simulink library "wcdma_lib"  (Simulink 6.0)
settings: Solver=ode45  SolverMode=SingleTasking  StartTime=0.0  StopTime=10.0  RelTol=1e-3
values from neighbouring files (symbols this model uses):
  allocationssc = [1 1 1 1 1 1 1 1 1 1 1 1 ... (960 elements, 64x15)]    [wcdma_allocationssc.mat]
  crcSize = str2num(Vals{idxCrcSize})    [wcdma_initmaskphlayer.m]    (also in wcdma_loadinitmuxandcoding.m = [16 12]; wcdma_loadinitphlayer.m = [16 12])
  errorCorr = (errorCorr>2)*2 + (errorCorr<3).*errorCorr    [wcdma_initmaskphlayer.m]    (also in wcdma_loadinitmuxandcoding.m = [2 2]; wcdma_loadinitphlayer.m = [2 2])
  i = [1:2:numSamp-1]'    [cdma2000_inttable.m]
  numBitsCodeWord = cond.*Zmin + not(cond).*numBitsCodeWord    [wcdma_concseg.m]    (also in wcdma_loadinitmuxandcoding.m = [260 122])
  numBitsFirstInt = numBitsRM + deltaNimax    [wcdma_initmaskphlayer.m]    (also in wcdma_loadinitmuxandcoding.m = [686 308])
  numBitsRF = numBitsFirstInt./(tti/10)    [wcdma_initmaskphlayer.m]    (also in wcdma_loadinitmuxandcoding.m = [343 77]; wcdma_loadinitphlayer.m = [343 77])
  numBitsTrCh = (trBlkSize+crcSize)*diag(numTrBlks)    [wcdma_concseg.m]    (also in wcdma_loadinitmuxandcoding.m = [260 112])
  numCodeWords = ceil(numBitsTrCh./Zmax(errorCorr+1))    [wcdma_concseg.m]    (also in wcdma_loadinitmuxandcoding.m = [1 1])
  numPadBits = (numBitsCodeWord.*numCodeWords)-numBitsTrCh    [wcdma_concseg.m]    (also in wcdma_loadinitmuxandcoding.m = [0 0])
  numPhCH = str2num(Vals{idxNumPhCH})    [wcdma_initmaskphlayer.m]    (also in wcdma_loadinitmuxandcoding.m = 1; wcdma_loadinitphlayer.m = 1)
  numTrBlks = trBlkSetSize./trBlkSize    [wcdma_concseg.m]    (also in wcdma_initmaskphlayer.m; wcdma_loadinitmuxandcoding.m = [1 1]; wcdma_loadinitphlayer.m = [1 1])
  overSampling = str2num(Vals{idxOverSampling})    [wcdma_initmaskphlayer.m]    (also in wcdma_initmaskspreadandmod.m; wcdma_loadinitphlayer.m = 8; wcdma_loadinitspreadandmod.m = 8)
  powerVector = str2num(Vals{idxPowerVector})    [wcdma_initmaskphlayer.m]    (also in wcdma_initmaskspreadandmod.m; wcdma_loadinitphlayer.m = [-5.5 -10 -15 -12 -12]; wcdma_loadinitspreadandmod.m = [-5.5 -10 -15 -12 -12])
  sprdFactor = wcdma_slotformattable(slotFormat+1,2)    [wcdma_checkparamstxant.m]    (also in wcdma_initmaskphlayer.m = slotformattable(slotFormat+1,2); wcdma_initmaskspreadandmod.m = slotformattable(slotFormat+1,2); wcdma_loadinitphlayer.m = 128; wcdma_loadinitspreadandmod.m = 128)
  tti = str2num(Vals{idxTti})    [wcdma_initmaskphlayer.m]    (also in wcdma_loadinitmuxandcoding.m = [20 40]; wcdma_loadinitphlayer.m = [20 40])
undefined symbols (not defined in the file or in its folder): hadamard, numSymbOut
libraries: wcdma_lib x122, dspsrcs4 x39, dspsigops x30, commseqgen2 x24, dspindex x20, dspbuff3 x19, dspmathops x16, simulink x10, dspsigattribs x7, commutil2 x6, dspmtrx3 x6, commblkintrlv2 x6
(part 2 of 3)

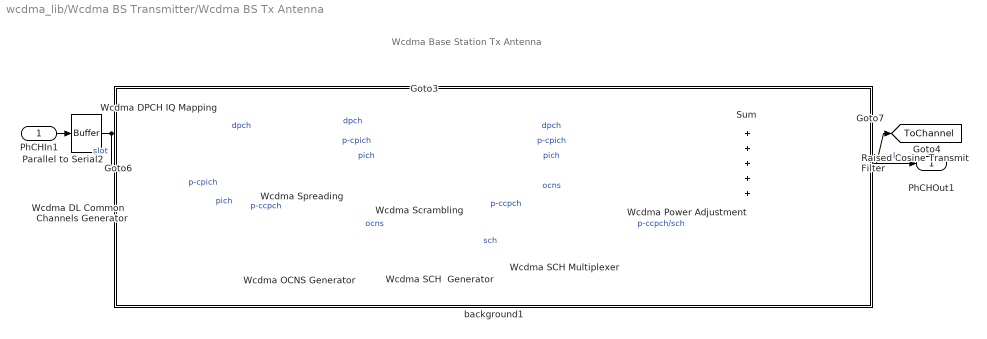
== system wcdma_lib/Wcdma BS Transmitter/Wcdma BS Tx Antenna ==
  note: Wcdma Base Station Tx Antenna
  PhCHIn1 : Inport  LatchInput=off
  Parallel to Serial2 : dspbuff3/Buffer  N=2*(numChipsOut/sprdFactor)  V=0  ic=0
  Raised Cosine Transmit Filter : commfilt2/Raised Cosine Transmit Filter  filtType=Square root  D=floor(numTapsRRC/(overSampling*2))  R=0.22  sampMode=Frame-based  N=overSampling  checkGain=User-specified  filterGain=sqrt(overSampling)  checkCoeff=off  variableName=rcTxFilt
  Sum : Sum  Inputs=+++++  SaturateOnIntegerOverflow=on  InputSameDT=on
  Wcdma DL Common  Channels Generator : wcdma_lib/Wcdma BS Transmitter/Wcdma DL Common  Channels Generator  antenna=1  numSymbOut=numChipsOut/256  st=1/15e3
  Wcdma DPCH IQ Mapping : wcdma_lib/Wcdma BS Transmitter/Wcdma DPCH IQ Mapping
  Wcdma OCNS Generator : wcdma_lib/Wcdma Sources/Wcdma OCNS Generator  sprdFactor=256  numSymbOut=numChipsOut/256  st=1/15e3
  Wcdma Power Adjustment : wcdma_lib/Wcdma BS Transmitter/Wcdma Power Adjustment  powerVector=powerVector
  Wcdma SCH  Generator : wcdma_lib/Wcdma Sources/Wcdma SCH  Generator  scrGroup=scrCode(1)  a_sch=1
  Wcdma SCH Multiplexer : wcdma_lib/Wcdma BS Transmitter/Wcdma SCH Multiplexer  numChipsOut=numChipsOut
  Wcdma Scrambling : wcdma_lib/Wcdma BS Transmitter/Wcdma Scrambling  scrCode=scrCode  numChipsOut=numChipsOut
  Wcdma Spreading : wcdma_lib/Wcdma BS Transmitter/Wcdma Spreading  sprdFactor=sprdFactor  dpchCode=dpchCode  codeVector=[0 4 1]  numChipsOut=numChipsOut
  background1 : Subsystem  EnableExecutionContextPropagation=on
      mask Display: disp('')
  PhCHOut1 : Outport
  tag scope: DPCH_Tx=global, DPCH_Tx_all=global, DPCH_Tx_sprd=global, ToChannel=global
  wires:
  Wcdma DPCH IQ Mapping/1 -> Wcdma Spreading/1  "dpch"
  Parallel to Serial2/1 -> Wcdma DPCH IQ Mapping/1, [DPCH_Tx]  "slot"
  Wcdma Spreading/3 -> Wcdma Scrambling/3  "pich"
  Wcdma Spreading/4 -> Wcdma Scrambling/4
  Wcdma DL Common  Channels Generator/1 -> Wcdma Spreading/2  "p-cpich"
  Wcdma Spreading/2 -> Wcdma Scrambling/2  "p-cpich"
  Wcdma Spreading/1 -> Wcdma Scrambling/1, [DPCH_Tx_sprd]  "dpch"
  Wcdma Scrambling/1 -> Wcdma Power Adjustment/1  "dpch"
  Wcdma Scrambling/2 -> Wcdma Power Adjustment/2  "p-cpich"
  Wcdma Scrambling/3 -> Wcdma Power Adjustment/3  "pich"
  Wcdma Power Adjustment/2 -> Sum/2
  Wcdma Power Adjustment/3 -> Sum/3
  Wcdma Power Adjustment/4 -> Sum/4
  Wcdma Power Adjustment/5 -> Sum/5
  Wcdma Scrambling/5 -> Wcdma Power Adjustment/5  "ocns"
  Wcdma Power Adjustment/1 -> Sum/1
  Wcdma SCH  Generator/1 -> Wcdma SCH Multiplexer/2  "sch"
  Wcdma Scrambling/4 -> Wcdma SCH Multiplexer/1  "p-ccpch"
  Wcdma SCH Multiplexer/1 -> Wcdma Power Adjustment/4  "p-ccpch/sch"
  Wcdma OCNS Generator/1 -> Wcdma Scrambling/5  "ocns"
  Wcdma DL Common  Channels Generator/2 -> Wcdma Spreading/3  "pich"
  Wcdma DL Common  Channels Generator/3 -> Wcdma Spreading/4  "p-ccpch"
  PhCHIn1/1 -> Parallel to Serial2/1
  Sum/1 -> [DPCH_Tx_all], Raised Cosine Transmit Filter/1
  Raised Cosine Transmit Filter/1 -> PhCHOut1/1, [ToChannel]  "l"

== system wcdma_lib/Wcdma BS Transmitter/Wcdma DL Common  Channels Generator ==
  P-CCPCH Generator : wcdma_lib/Wcdma Sources/Channel Generator  rndSeed=98765  initDelay=0  numSymbOut=numSymbOut  st=st
  P-CPICH Generator : wcdma_lib/Wcdma Sources/P-CPICH Generator  antenna=antenna  numSymbOut=numSymbOut  st=st
  PICH Generator : wcdma_lib/Wcdma Sources/Channel Generator  rndSeed=12345  initDelay=0  numSymbOut=numSymbOut  st=st
  cP-CPICH : Outport
  cPICH : Outport  Port=2
  cP-CCPCH : Outport  Port=3
  wires:
  P-CPICH Generator/1 -> cP-CPICH/1
  PICH Generator/1 -> cPICH/1
  P-CCPCH Generator/1 -> cP-CCPCH/1

== system wcdma_lib/Wcdma BS Transmitter/Wcdma DPCH IQ Mapping ==
  DPCH : Inport  LatchInput=off
  Bit to Integer Converter : commutil2/Bit to Integer Converter  nbits=2
  Data Mapper : commutil2/Data Mapper  MapMode=User Defined  M=4  MapVec=[0 3 1 2]
  QPSK Modulator Baseband : commdigbbndpm2/QPSK Modulator Baseband  InType=Integer  Enc=Binary  Ph=pi/4  numSamp=1
  cDPCH : Outport
  wires:
  Bit to Integer Converter/1 -> Data Mapper/1
  Data Mapper/1 -> QPSK Modulator Baseband/1
  DPCH/1 -> Bit to Integer Converter/1
  QPSK Modulator Baseband/1 -> cDPCH/1

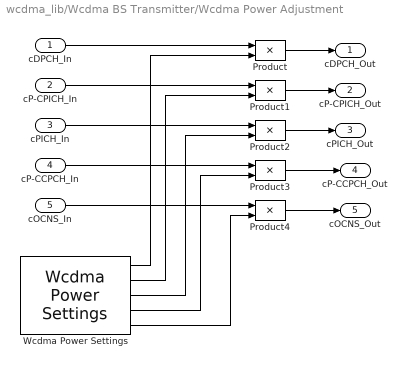
== system wcdma_lib/Wcdma BS Transmitter/Wcdma Power Adjustment ==
  cDPCH_In : Inport  LatchInput=off
  cP-CPICH_In : Inport  Port=2  LatchInput=off
  cPICH_In : Inport  Port=3  LatchInput=off
  cP-CCPCH_In : Inport  Port=4  LatchInput=off
  cOCNS_In : Inport  Port=5  LatchInput=off
  Product{,1..4} (5 alike) : Product  SaturateOnIntegerOverflow=on  InputSameDT=on
  Wcdma Power Settings : wcdma_lib/Wcdma BS Transmitter/Wcdma Power Settings  powerVector=powerVector
  cDPCH_Out : Outport
  cP-CPICH_Out : Outport  Port=2
  cPICH_Out : Outport  Port=3
  cP-CCPCH_Out : Outport  Port=4
  cOCNS_Out : Outport  Port=5
  wires:
  cDPCH_In/1 -> Product/1
  Product/1 -> cDPCH_Out/1
  cP-CPICH_In/1 -> Product1/1
  Product1/1 -> cP-CPICH_Out/1
  cPICH_In/1 -> Product2/1
  Product2/1 -> cPICH_Out/1
  cP-CCPCH_In/1 -> Product3/1
  Product3/1 -> cP-CCPCH_Out/1
  cOCNS_In/1 -> Product4/1
  Product4/1 -> cOCNS_Out/1
  Wcdma Power Settings/1 -> Product/2
  Wcdma Power Settings/2 -> Product1/2
  Wcdma Power Settings/3 -> Product2/2
  Wcdma Power Settings/4 -> Product3/2
  Wcdma Power Settings/5 -> Product4/2

== system wcdma_lib/Wcdma BS Transmitter/Wcdma Power Settings ==
  Constant : Constant  Value=powerVector(1:4)'  VectorParams1D=off
  Constant1 : Constant
  Multiport Selector1 : dspindex/Multiport Selector  rowsOrCols=Rows  idxCellArray={1,2,3, 4}  idxErrMode=Clip and Warn
  Sum : Sum  Inputs=+  SaturateOnIntegerOverflow=on  InputSameDT=on
  Sum1 : Sum  Inputs=|+-  SaturateOnIntegerOverflow=on  InputSameDT=on
  dB-Linear Conversion : wcdma_lib/Wcdma Common/dB-Linear Conversion
  log1 : Math  Operator=sqrt  SaturateOnIntegerOverflow=on
  log5 : Math  Operator=sqrt  SaturateOnIntegerOverflow=on
  DPCH_Ec : Outport
  P-CPICH_Ec : Outport  Port=2
  PICH_Ec : Outport  Port=3
  P-CCPCH_Ec/SCH_Ec : Outport  Port=4
  OCNS_Ec : Outport  Port=5
  wires:
  dB-Linear Conversion/1 -> log1/1, Sum/1
  log5/1 -> OCNS_Ec/1
  Sum1/1 -> log5/1
  Sum/1 -> Sum1/2
  Constant1/1 -> Sum1/1
  Constant/1 -> dB-Linear Conversion/1
  Multiport Selector1/1 -> DPCH_Ec/1
  Multiport Selector1/2 -> P-CPICH_Ec/1
  log1/1 -> Multiport Selector1/1
  Multiport Selector1/3 -> PICH_Ec/1
  Multiport Selector1/4 -> P-CCPCH_Ec/SCH_Ec/1

== system wcdma_lib/Wcdma BS Transmitter/Wcdma SCH Multiplexer ==
  P-CCPCH_In : Inport  LatchInput=off
  SCH_In : Inport  Port=2  LatchInput=off
  DSP Constant1 : dspsrcs4/DSP Constant  Value=numSymbOut  InterpretAs1D=off  SampleMode=Discrete  Ts=numSymbOut/15e3  FramebasedOutput=off
  DSP Constant2 : dspsrcs4/DSP Constant  Value=[1:numSymbOut]  InterpretAs1D=off  SampleMode=Discrete  Ts=numSymbOut/15e3  FramebasedOutput=off
  Matrix Concatenation : simulink/Math Operations/Matrix Concatenation  numInports=2  catMethod=Horizontal
  Pulse Generator : DiscretePulseGenerator  Period=10/numSymbOut  SampleTime=numSymbOut/15e3
  Reshape : simulink/Math Operations/Reshape  OutputDimensionality=Customize  OutputDimensions=[256,numSymbOut]
  Reshape1 : simulink/Math Operations/Reshape  OutputDimensionality=Customize  OutputDimensions=[256*numSymbOut,1]
  Switch : Switch  Threshold=0.5  InputSameDT=on
  Variable Selector : dspindex/Variable Selector  rowsOrCols=Columns  IdxMode=Variable  Elements=[1 3]  ZerOneIdxMode=One-based  errmode=Clip Index
  Variable Selector1 : dspindex/Variable Selector  rowsOrCols=Columns  IdxMode=Variable  Elements=[1 3]  ZerOneIdxMode=One-based  errmode=Clip Index
  cSCH/PCCPCH : Outport
  wires:
  Pulse Generator/1 -> Switch/2
  Reshape1/1 -> Switch/1
  Switch/1 -> cSCH/PCCPCH/1
  DSP Constant2/1 -> Variable Selector1/2
  Variable Selector1/1 -> Reshape1/1
  Matrix Concatenation/1 -> Variable Selector1/1
  SCH_In/1 -> Matrix Concatenation/1
  Variable Selector/1 -> Matrix Concatenation/2
  DSP Constant1/1 -> Variable Selector/2
  Reshape/1 -> Variable Selector/1
  P-CCPCH_In/1 -> Switch/3, Reshape/1

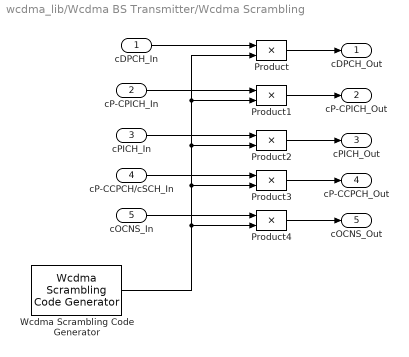
== system wcdma_lib/Wcdma BS Transmitter/Wcdma Scrambling ==
  cDPCH_In : Inport  LatchInput=off
  cP-CPICH_In : Inport  Port=2  LatchInput=off
  cPICH_In : Inport  Port=3  LatchInput=off
  cP-CCPCH/cSCH_In : Inport  Port=4  LatchInput=off
  cOCNS_In : Inport  Port=5  LatchInput=off
  Product{,1..4} (5 alike) : Product  SaturateOnIntegerOverflow=on  InputSameDT=on
  Wcdma Scrambling Code Generator : wcdma_lib/Wcdma Sources/Wcdma Scrambling Code Generator  scrCode=scrCode  chipRate=3.84e6  numChipsOut=numChipsOut
  cDPCH_Out : Outport
  cP-CPICH_Out : Outport  Port=2
  cPICH_Out : Outport  Port=3
  cP-CCPCH_Out : Outport  Port=4
  cOCNS_Out : Outport  Port=5
  wires:
  cDPCH_In/1 -> Product/1
  Product/1 -> cDPCH_Out/1
  cP-CPICH_In/1 -> Product1/1
  Product1/1 -> cP-CPICH_Out/1
  cPICH_In/1 -> Product2/1
  Product2/1 -> cPICH_Out/1
  cP-CCPCH/cSCH_In/1 -> Product3/1
  Product3/1 -> cP-CCPCH_Out/1
  cOCNS_In/1 -> Product4/1
  Product4/1 -> cOCNS_Out/1
  Wcdma Scrambling Code Generator/1 -> Product/2, Product1/2, Product2/2, Product3/2, Product4/2

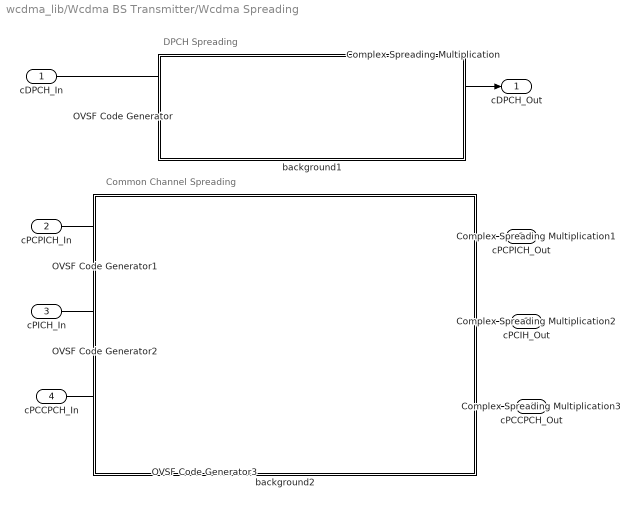
== system wcdma_lib/Wcdma BS Transmitter/Wcdma Spreading ==
  note: DPCH Spreading
  note: Common Channel Spreading
  cDPCH_In : Inport  LatchInput=off
  cPCPICH_In : Inport  Port=2  LatchInput=off
  cPICH_In : Inport  Port=3  LatchInput=off
  cPCCPCH_In : Inport  Port=4  LatchInput=off
  Complex Spreading Multiplication : wcdma_lib/Wcdma BS Transmitter/Complex Spreading Multiplication  sprdFactor=sprdFactor
  Complex Spreading Multiplication1 : wcdma_lib/Wcdma BS Transmitter/Complex Spreading Multiplication  sprdFactor=256
  Complex Spreading Multiplication2 : wcdma_lib/Wcdma BS Transmitter/Complex Spreading Multiplication  sprdFactor=256
  Complex Spreading Multiplication3 : wcdma_lib/Wcdma BS Transmitter/Complex Spreading Multiplication  sprdFactor=256
  OVSF Code Generator : commseqgen2/OVSF Code Generator  spreadFact=sprdFactor  index=dpchCode  ts=(numChipsOut/256)/15e3  frameBased=on  sampPerFrame=numChipsOut
  OVSF Code Generator1 : commseqgen2/OVSF Code Generator  spreadFact=256  index=codeVector(1)  ts=(numChipsOut/256)/15e3  frameBased=on  sampPerFrame=numChipsOut
  OVSF Code Generator2 : commseqgen2/OVSF Code Generator  spreadFact=256  index=codeVector(2)  ts=(numChipsOut/256)/15e3  frameBased=on  sampPerFrame=numChipsOut
  OVSF Code Generator3 : commseqgen2/OVSF Code Generator  spreadFact=256  index=codeVector(3)  ts=(numChipsOut/256)/15e3  frameBased=on  sampPerFrame=numChipsOut
  background1 : Subsystem  EnableExecutionContextPropagation=on
      mask Display: disp('')
  background2 : Subsystem  EnableExecutionContextPropagation=on
      mask Display: disp('')
  cDPCH_Out : Outport
  cPCPICH_Out : Outport  Port=2
  cPCIH_Out : Outport  Port=3
  cPCCPCH_Out : Outport  Port=4
  wires:
  Complex Spreading Multiplication3/1 -> cPCCPCH_Out/1
  cPCCPCH_In/1 -> Complex Spreading Multiplication3/1
  Complex Spreading Multiplication2/1 -> cPCIH_Out/1
  cPICH_In/1 -> Complex Spreading Multiplication2/1
  Complex Spreading Multiplication1/1 -> cPCPICH_Out/1
  cPCPICH_In/1 -> Complex Spreading Multiplication1/1
  Complex Spreading Multiplication/1 -> cDPCH_Out/1
  cDPCH_In/1 -> Complex Spreading Multiplication/1
  OVSF Code Generator/1 -> Complex Spreading Multiplication/2
  OVSF Code Generator1/1 -> Complex Spreading Multiplication1/2
  OVSF Code Generator2/1 -> Complex Spreading Multiplication2/2
  OVSF Code Generator3/1 -> Complex Spreading Multiplication3/2

== system wcdma_lib/Wcdma Channel Model/AWGN ==
  ChIn : Inport  LatchInput=off
  AWGN Channel : commchan2/AWGN Channel  seed=1237  noiseMode="Signal to noise ratio  (Es/No)"  EsNodB=snrdB  SNRdB=snrdB  Ps=1  Tsym=1/3.84e6  variance=1
  ChOut : Outport
  wires:
  AWGN Channel/1 -> ChOut/1
  ChIn/1 -> AWGN Channel/1

== system wcdma_lib/Wcdma Channel Model/Multipath+AWGN ==
  ChIn : Inport  LatchInput=off
  AWGN Channel : commchan2/AWGN Channel  seed=1237  noiseMode="Signal to noise ratio  (Es/No)"  EsNodB=snrdB  SNRdB=snrdB  Ps=1  Tsym=1/3.84e6  variance=1
  Multipath Rayleigh Fading Channel : commchan2/Multipath Rayleigh Fading Channel  Fd=dopplerFreq  simTs=1/(overSampling*3.84e6)  delayVec=fingerPhases  gainVecdB=fingerPowers  normGain=off  Seed=12345
  ChOut : Outport
  wires:
  Multipath Rayleigh Fading Channel/1 -> AWGN Channel/1
  ChIn/1 -> Multipath Rayleigh Fading Channel/1
  AWGN Channel/1 -> ChOut/1

== system wcdma_lib/Wcdma Channel Model/No Channel ==
  ChIn : Inport  LatchInput=off
  ChOut : Outport
  wires:
  ChIn/1 -> ChOut/1

== system wcdma_lib/Wcdma Channel Model/Wcdma Channel Models ==
  ChIn : Inport  LatchInput=off
  AWGN : wcdma_lib/Wcdma Channel Model/AWGN
  ChOut : Outport
  wires:
  ChIn/1 -> AWGN/1
  AWGN/1 -> ChOut/1

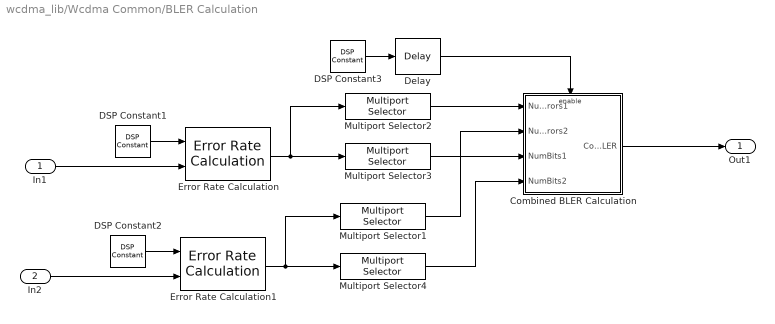
== system wcdma_lib/Wcdma Common/BLER Calculation ==
  In1 : Inport  LatchInput=off
  In2 : Inport  Port=2  LatchInput=off
  Combined BLER Calculation : Subsystem  TreatAsAtomicUnit=on  EnableExecutionContextPropagation=on
      mask Display: disp('Combined\nBLER\nCalculation');
  DSP Constant1 : dspsrcs4/DSP Constant  Value=0  SampleMode=Discrete  discreteOutput=Sample-based  continuousOutput=Sample-based  sampTime=tti(1)*(1e-3)  framePeriod=tti(1)*(1e-3)  dataType=Inherit from 'Constant value'  wordLen=16  udDataType=sfix(16)  fracBitsMode=Best precision  numFracBits=15  InterpretAs1D=off  Ts=tti(1)*(1e-3)  FramebasedOutput=off
  DSP Constant2 : dspsrcs4/DSP Constant  Value=0  SampleMode=Discrete  discreteOutput=Sample-based  continuousOutput=Sample-based  sampTime=tti(2)*(1e-3)  framePeriod=tti(2)*(1e-3)  dataType=Inherit from 'Constant value'  wordLen=16  udDataType=sfix(16)  fracBitsMode=Best precision  numFracBits=15  InterpretAs1D=off  Ts=tti(2)*(1e-3)  FramebasedOutput=off
  DSP Constant3 : dspsrcs4/DSP Constant  Value=1  SampleMode=Discrete  discreteOutput=Sample-based  continuousOutput=Sample-based  sampTime=tti(i)*(1e-3)  framePeriod=tti(i)*(1e-3)  dataType=Inherit from 'Constant value'  wordLen=16  udDataType=sfix(16)  fracBitsMode=Best precision  numFracBits=15  InterpretAs1D=off  Ts=tti(i)*(1e-3)  FramebasedOutput=off
  Delay : dspsigops/Delay  dly_unit=Samples  delay=minNumTrBlksDelay  ic_detail=off  dif_ic_for_ch=off  dif_ic_for_dly=off  ic=0  reset_popup=None
  Error Rate Calculation : commsink2/Error Rate Calculation  N=0  st_delay=numTrBlksDelay(1)  cp_mode=Entire frame  subframe=[]  PMode=Port  WsName=ErrorVec  RsMode2=off  stop=off  numErr=100  maxBits=1e6
  Error Rate Calculation1 : commsink2/Error Rate Calculation  N=0  st_delay=numTrBlksDelay(2)  cp_mode=Entire frame  subframe=[]  PMode=Port  WsName=ErrorVec  RsMode2=off  stop=off  numErr=100  maxBits=1e6
  Multiport Selector1 : dspindex/Multiport Selector  rowsOrCols=Rows  idxCellArray=2  idxErrMode=Clip Index
  Multiport Selector2 : dspindex/Multiport Selector  rowsOrCols=Rows  idxCellArray=2  idxErrMode=Clip Index
  Multiport Selector3 : dspindex/Multiport Selector  rowsOrCols=Rows  idxCellArray=3  idxErrMode=Clip Index
  Multiport Selector4 : dspindex/Multiport Selector  rowsOrCols=Rows  idxCellArray=3  idxErrMode=Clip Index
  Out1 : Outport
  wires:
  Combined BLER Calculation/1(Combined BLER) -> Out1/1
  In1/1 -> Error Rate Calculation/2
  Multiport Selector3/1 -> Combined BLER Calculation/3(NumBits1)
  Multiport Selector2/1 -> Combined BLER Calculation/1(NumErrors1)
  Error Rate Calculation/1 -> Multiport Selector2/1, Multiport Selector3/1
  DSP Constant1/1 -> Error Rate Calculation/1
  In2/1 -> Error Rate Calculation1/2
  Multiport Selector4/1 -> Combined BLER Calculation/4(NumBits2)
  Multiport Selector1/1 -> Combined BLER Calculation/2(NumErrors2)
  Error Rate Calculation1/1 -> Multiport Selector4/1, Multiport Selector1/1
  DSP Constant2/1 -> Error Rate Calculation1/1
  DSP Constant3/1 -> Delay/1
  Delay/1 -> Combined BLER Calculation/Enable

== system wcdma_lib/Wcdma Common/Complex Unipolar to Bipolar  ==
  In1 : Inport  LatchInput=off
  Constant : Constant  Value=M-1
  Gain : Gain  Gain=2
  Inherit Complexity : dspsigattribs/Inherit Complexity
  Polarity : Gain  Gain=pole
  Probe : Probe  ProbeWidth=off  ProbeSampleTime=off
  Product : Product  SaturateOnIntegerOverflow=on  InputSameDT=on
  Real-Imag to Complex : RealImagToComplex
  Sum : Sum  Inputs=|+-  InputSameDT=on
  Out1 : Outport
  wires:
  Real-Imag to Complex/1 -> Sum/2
  Constant/1 -> Real-Imag to Complex/1, Product/1
  Sum/1 -> Polarity/1
  Polarity/1 -> Inherit Complexity/1
  Gain/1 -> Sum/1
  In1/1 -> Gain/1, Probe/1, Inherit Complexity/2
  Product/1 -> Real-Imag to Complex/2
  Probe/1 -> Product/2
  Inherit Complexity/1 -> Out1/1

== system wcdma_lib/Wcdma Common/Complex  Bipolar to Unipolar ==
  In2 : Inport  LatchInput=off
  Constant1 : Constant  Value=M-1
  Gain1 : Gain  Gain=0.5
  Inherit Complexity : dspsigattribs/Inherit Complexity
  Polarity : Gain  Gain=pole
  Probe : Probe  ProbeWidth=off  ProbeSampleTime=off
  Product : Product  SaturateOnIntegerOverflow=on  InputSameDT=on
  Real-Imag to Complex : RealImagToComplex
  Sum1 : Sum  Inputs=|++  InputSameDT=on
  Out2 : Outport
  wires:
  Real-Imag to Complex/1 -> Sum1/2
  Constant1/1 -> Real-Imag to Complex/1, Product/1
  Sum1/1 -> Gain1/1
  In2/1 -> Polarity/1, Probe/1, Inherit Complexity/2
  Product/1 -> Real-Imag to Complex/2
  Probe/1 -> Product/2
  Polarity/1 -> Sum1/1
  Gain1/1 -> Inherit Complexity/1
  Inherit Complexity/1 -> Out2/1

== system wcdma_lib/Wcdma Common/Energy Measurement ==
  cIn : Inport  LatchInput=off
  Frame Status Conversion : dspsigattribs/Frame Status Conversion  growRefPort=off  outframe=Frame-based
  Matrix Multiply : dspmtrx3/Matrix Multiply  numInputPorts=2  OptimizationLevel=None
  Transpose : dspmtrx3/Transpose  Hermitian=on
  Out : Outport
  wires:
  cIn/1 -> Transpose/1, Matrix Multiply/2
  Matrix Multiply/1 -> Out/1
  Transpose/1 -> Frame Status Conversion/1
  Frame Status Conversion/1 -> Matrix Multiply/1

== system wcdma_lib/Wcdma Common/Hadamard Matrix ==
  Hadamard Matrix : dspsrcs4/DSP Constant  Value=hadamard(2^order)  InterpretAs1D=off  SampleMode=Discrete  Ts=0.01/15  FramebasedOutput=on
  Out1 : Outport
  wires:
  Hadamard Matrix/1 -> Out1/1

== system wcdma_lib/Wcdma Common/Low Pass Filter ==
  In1 : Inport  LatchInput=off
  Digital Filter : dsparch4/Digital Filter  TypePopup=FIR (all zeros)  IIRFiltStruct=Direct form II transposed  AllPoleFiltStruct=Direct form  FIRFiltStruct=Direct form  CoeffSource=Specify via dialog  NumCoeffs=h  DenCoeffs=[1 0.1]  BiQuadCoeffs=[1 0.3 0.4 1 0.1 0.2]  LatticeCoeffs=[0.2 0.4]  denIgnore=on  FiltPerSampPopup=One filter per frame  IC=outputBufInitCond  ICnum=0  ICden=0
  Out1 : Outport
  wires:
  In1/1 -> Digital Filter/1
  Digital Filter/1 -> Out1/1

== system wcdma_lib/Wcdma Common/Normalize Ec ==
  In1 : Inport  LatchInput=off
  DSP Constant : dspsrcs4/DSP Constant  Value=1e-6  InterpretAs1D=on  SampleMode=Discrete  Ts=1  FramebasedOutput=off
  Math Function : Math  Operator=sqrt  SaturateOnIntegerOverflow=on
  Power  Measurement : Subsystem  EnableExecutionContextPropagation=on
      mask Display: disp('Power\nMeasurement')
  Product : Product  Inputs=*/  SaturateOnIntegerOverflow=on  InputSameDT=on
  Sum : Sum  Inputs=|++  SaturateOnIntegerOverflow=on  InputSameDT=on
  Out1 : Outport
  wires:
  Power  Measurement/1(Power) -> Sum/1
  DSP Constant/1 -> Sum/2
  Sum/1 -> Math Function/1
  In1/1 -> Power  Measurement/1(cIn), Product/1
  Product/1 -> Out1/1
  Math Function/1 -> Product/2

== system wcdma_lib/Wcdma Common/dB-Linear Conversion ==
  Power_dB : Inport  LatchInput=off
  Gain1 : Gain  Gain=1/10  SaturateOnIntegerOverflow=on
  log1 : Math  Operator=10^u  SaturateOnIntegerOverflow=on
  Power_linear : Outport
  wires:
  Power_dB/1 -> Gain1/1
  Gain1/1 -> log1/1
  log1/1 -> Power_linear/1

== system wcdma_lib/Wcdma Multiplexing and Channel Coding/1st DeInterleaver ==
  TrChIn1 : Inport  LatchInput=off
  TrChIn2 : Inport  Port=2  LatchInput=off
  Wcdma 1st DeInterleaver : wcdma_lib/Wcdma Multiplexing and Channel Coding/Wcdma 1st DeInterleaver  numBits=numBitsFirstInt(1)  tti=tti(1)
  Wcdma 1st DeInterleaver1 : wcdma_lib/Wcdma Multiplexing and Channel Coding/Wcdma 1st DeInterleaver  numBits=numBitsFirstInt(2)  tti=tti(2)
  TrChOut1 : Outport
  TrChOut2 : Outport  Port=2
  wires:
  Wcdma 1st DeInterleaver1/1 -> TrChOut2/1
  Wcdma 1st DeInterleaver/1 -> TrChOut1/1
  TrChIn2/1 -> Wcdma 1st DeInterleaver1/1
  TrChIn1/1 -> Wcdma 1st DeInterleaver/1

== system wcdma_lib/Wcdma Multiplexing and Channel Coding/1st Interleaver ==
  TrChIn1 : Inport  LatchInput=off
  TrChIn2 : Inport  Port=2  LatchInput=off
  Wcdma 1st Interleaver : wcdma_lib/Wcdma Multiplexing and Channel Coding/Wcdma 1st Interleaver  numBits=numBitsFirstInt(1)  tti=tti(1)
  Wcdma 1st Interleaver1 : wcdma_lib/Wcdma Multiplexing and Channel Coding/Wcdma 1st Interleaver  numBits=numBitsFirstInt(2)  tti=tti(2)
  TrChOut1 : Outport
  TrChOut2 : Outport  Port=2
  wires:
  TrChIn1/1 -> Wcdma 1st Interleaver/1
  TrChIn2/1 -> Wcdma 1st Interleaver1/1
  Wcdma 1st Interleaver/1 -> TrChOut1/1
  Wcdma 1st Interleaver1/1 -> TrChOut2/1

== system wcdma_lib/Wcdma Multiplexing and Channel Coding/2nd DeInterleaver ==
  PhChIn1 : Inport  LatchInput=off
  Wcdma 2nd DeInterleaver : wcdma_lib/Wcdma Multiplexing and Channel Coding/Wcdma 2nd DeInterleaver  numBits=sum(numBitsRF)/numPhCH
  PhChOut1 : Outport
  wires:
  PhChIn1/1 -> Wcdma 2nd DeInterleaver/1
  Wcdma 2nd DeInterleaver/1 -> PhChOut1/1

== system wcdma_lib/Wcdma Multiplexing and Channel Coding/2nd Interleaver ==
  PhChIn1 : Inport  LatchInput=off
  Wcdma 2nd Interleaver : wcdma_lib/Wcdma Multiplexing and Channel Coding/Wcdma 2nd Interleaver  numBits=sum(numBitsRF)/numPhCH
  PhChOut1 : Outport
  wires:
  Wcdma 2nd Interleaver/1 -> PhChOut1/1
  PhChIn1/1 -> Wcdma 2nd Interleaver/1

== system wcdma_lib/Wcdma Multiplexing and Channel Coding/CRC Calculation ==
  TrChIn1 : Inport  LatchInput=off
  TrChIn2 : Inport  Port=2  LatchInput=off
  Wcdma CRC Generator : wcdma_lib/Wcdma Multiplexing and Channel Coding/Wcdma CRC Generator  bits=crcSize(1)  iniStates=0  dataFrames=numTrBlks(1)
  Wcdma CRC Generator1 : wcdma_lib/Wcdma Multiplexing and Channel Coding/Wcdma CRC Generator  bits=crcSize(2)  iniStates=0  dataFrames=numTrBlks(2)
  TrChOut1 : Outport
  TrChOut2 : Outport  Port=2
  wires:
  TrChIn1/1 -> Wcdma CRC Generator/1
  TrChIn2/1 -> Wcdma CRC Generator1/1
  Wcdma CRC Generator/1 -> TrChOut1/1
  Wcdma CRC Generator1/1 -> TrChOut2/1

== system wcdma_lib/Wcdma Multiplexing and Channel Coding/Channel Decoding ==
  TrChIn1 : Inport  LatchInput=off
  TrChIn2 : Inport  Port=2  LatchInput=off
  Wcdma Channel Decoding : wcdma_lib/Wcdma Multiplexing and Channel Coding/Wcdma Channel Decoding  errorCorr=errorCorr(1)  numBitsCodeWord=numBitsCodeWord(1)  numCodeWords=numCodeWords(1)  tti=tti(1)
  Wcdma Channel Decoding1 : wcdma_lib/Wcdma Multiplexing and Channel Coding/Wcdma Channel Decoding  errorCorr=errorCorr(2)  numBitsCodeWord=numBitsCodeWord(2)  numCodeWords=numCodeWords(2)  tti=tti(2)
  CodeWordOut1 : Outport
  CodeWordOut2 : Outport  Port=2
  wires:
  TrChIn2/1 -> Wcdma Channel Decoding1/1
  TrChIn1/1 -> Wcdma Channel Decoding/1
  Wcdma Channel Decoding/1 -> CodeWordOut1/1
  Wcdma Channel Decoding1/1 -> CodeWordOut2/1

== system wcdma_lib/Wcdma Multiplexing and Channel Coding/Channel Encoding ==
  CodeWordIn1 : Inport  LatchInput=off
  CodeWordIn2 : Inport  Port=2  LatchInput=off
  Wcdma Channel Encoding : wcdma_lib/Wcdma Multiplexing and Channel Coding/Wcdma Channel Encoding  errorCorr=errorCorr(1)  numBitsCodeWord=numBitsCodeWord(1)  numCodeWords=numCodeWords(1)  tti=tti(1)
  Wcdma Channel Encoding1 : wcdma_lib/Wcdma Multiplexing and Channel Coding/Wcdma Channel Encoding  errorCorr=errorCorr(2)  numBitsCodeWord=numBitsCodeWord(2)  numCodeWords=numCodeWords(2)  tti=tti(2)
  TrChOut1 : Outport
  TrChOut2 : Outport  Port=2
  wires:
  CodeWordIn1/1 -> Wcdma Channel Encoding/1
  CodeWordIn2/1 -> Wcdma Channel Encoding1/1
  Wcdma Channel Encoding/1 -> TrChOut1/1
  Wcdma Channel Encoding1/1 -> TrChOut2/1

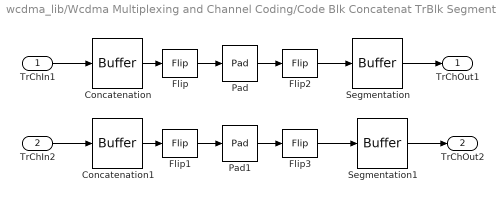
== system wcdma_lib/Wcdma Multiplexing and Channel Coding/Code Blk Concatenat TrBlk Segment ==
  TrChIn1 : Inport  LatchInput=off
  TrChIn2 : Inport  Port=2  LatchInput=off
  Concatenation : dspbuff3/Buffer  N=numBitsTrCh(1)+numPadBits(1)  V=0  ic=0
  Concatenation1 : dspbuff3/Buffer  N=numBitsTrCh(2)+numPadBits(2)  V=0  ic=0
  Flip{,1..3} (4 alike) : dspindex/Flip  dim=Columns
  Pad : dspsigops/Pad  padVal=0  padAlong=Columns  numOutRows=numBitsTrCh(1)  numOutCols=1  trunc_flag=None
  Pad1 : dspsigops/Pad  padVal=0  padAlong=Columns  numOutRows=numBitsTrCh(2)  numOutCols=1  trunc_flag=None
  Segmentation : dspbuff3/Buffer  N=(trBlkSize(1)+crcSize(1))*numTrBlks(1)  V=0  ic=0
  Segmentation1 : dspbuff3/Buffer  N=(trBlkSize(2)+crcSize(2))*numTrBlks(2)  V=0  ic=0
  TrChOut1 : Outport
  TrChOut2 : Outport  Port=2
  wires:
  TrChIn2/1 -> Concatenation1/1
  TrChIn1/1 -> Concatenation/1
  Segmentation/1 -> TrChOut1/1
  Segmentation1/1 -> TrChOut2/1
  Concatenation/1 -> Flip/1
  Concatenation1/1 -> Flip1/1
  Flip/1 -> Pad/1
  Flip1/1 -> Pad1/1
  Pad/1 -> Flip2/1
  Pad1/1 -> Flip3/1
  Flip2/1 -> Segmentation/1
  Flip3/1 -> Segmentation1/1

== system wcdma_lib/Wcdma Multiplexing and Channel Coding/PhCh Concatenation ==
  CCTrCH1 : Inport  LatchInput=off
  Matrix Concatenation : simulink/Math Operations/Matrix Concatenation  numInports=numPhCH  catMethod=Vertical
  PhCh1 : Outport
  wires:
  Matrix Concatenation/1 -> PhCh1/1
  CCTrCH1/1 -> Matrix Concatenation/1

== system wcdma_lib/Wcdma Multiplexing and Channel Coding/PhCh Segmentation ==
  CCTrCH1 : Inport  LatchInput=off
  Demux : Demux  Outputs=numPhCH
  PhCh1 : Outport
  wires:
  CCTrCH1/1 -> Demux/1
  Demux/1 -> PhCh1/1

== system wcdma_lib/Wcdma Multiplexing and Channel Coding/Radio Frame  Concatenation ==
  CCTrCH1 : Inport  LatchInput=off
  Buffer : dspbuff3/Buffer  N=numBits(1)  V=0  ic=0
  Buffer1 : dspbuff3/Buffer  N=numBits(2)  V=0  ic=0
  Delay : dspsigops/Delay  dly_unit=Samples  delay=(((tti(1)-20)/10)*numBitsRF(1))*checkDelay*(tti(1)~=10)  ic_detail=off  dif_ic_for_ch=off  dif_ic_for_dly=off  ic=0  reset_popup=None
  Delay1 : dspsigops/Delay  dly_unit=Samples  delay=(((tti(2)-20)/10)*numBitsRF(2))*checkDelay*(tti(2)~=10)  ic_detail=off  dif_ic_for_ch=off  dif_ic_for_dly=off  ic=0  reset_popup=None
  Multiport Selector : dspindex/Multiport Selector  rowsOrCols=Rows  idxCellArray={[1:numBitsRF(1)] [numBitsRF(1)+1:numBitsRF(1)+numBitsRF(2)]}  idxErrMode=Clip Index
  TrChOut1 : Outport
  TrChOut2 : Outport  Port=2
  wires:
  Multiport Selector/2 -> Delay1/1  "Radio Frame"
  Multiport Selector/1 -> Delay/1  "Radio Frame"
  CCTrCH1/1 -> Multiport Selector/1  "CCTrCH"
  Buffer/1 -> TrChOut1/1  "Transport Channel"
  Buffer1/1 -> TrChOut2/1  "Transport Channel"
  Delay/1 -> Buffer/1
  Delay1/1 -> Buffer1/1

== system wcdma_lib/Wcdma Multiplexing and Channel Coding/Radio Frame  Segmentation ==
  TrChIn1 : Inport  LatchInput=off
  TrChIn2 : Inport  Port=2  LatchInput=off
  Buffer : dspbuff3/Buffer  N=numBitsRF(1)  V=0  ic=0
  Buffer1 : dspbuff3/Buffer  N=numBitsRF(2)  V=0  ic=0
  Matrix Concatenation : simulink/Math Operations/Matrix Concatenation  numInports=2  catMethod=Vertical
  CCTrCh1 : Outport
  wires:
  Matrix Concatenation/1 -> CCTrCh1/1  "CCTrCH"
  TrChIn1/1 -> Buffer/1  "Transport Channel"
  TrChIn2/1 -> Buffer1/1  "Transport Channel"
  Buffer1/1 -> Matrix Concatenation/2  "Radio Frame"
  Buffer/1 -> Matrix Concatenation/1  "Radio Frame"

== system wcdma_lib/Wcdma Multiplexing and Channel Coding/Rate DeMatching ==
  TrChIn1 : Inport  LatchInput=off
  TrChIn2 : Inport  Port=2  LatchInput=off
  Wcdma Rate Matching : wcdma_lib/Wcdma Multiplexing and Channel Coding/Wcdma Rate Matching  idxTrCh=1  numBits=numBitsRM  RMAttribute=RMAttribute  tti=tti  errorCorr=errorCorr  posTrCh=posTrCh  slotFormat=slotFormat  numPhCH=numPhCH  checkRM=on
  Wcdma Rate Matching1 : wcdma_lib/Wcdma Multiplexing and Channel Coding/Wcdma Rate Matching  idxTrCh=2  numBits=numBitsRM  RMAttribute=RMAttribute  tti=tti  errorCorr=errorCorr  posTrCh=posTrCh  slotFormat=slotFormat  numPhCH=numPhCH  checkRM=on
  TrChOut1 : Outport
  TrChOut2 : Outport  Port=2
  wires:
  TrChIn1/1 -> Wcdma Rate Matching/1
  TrChIn2/1 -> Wcdma Rate Matching1/1
  Wcdma Rate Matching/1 -> TrChOut1/1
  Wcdma Rate Matching1/1 -> TrChOut2/1

== system wcdma_lib/Wcdma Multiplexing and Channel Coding/Rate Matching ==
  TrChIn1 : Inport  LatchInput=off
  TrChIn2 : Inport  Port=2  LatchInput=off
  Wcdma Rate Matching : wcdma_lib/Wcdma Multiplexing and Channel Coding/Wcdma Rate Matching  idxTrCh=1  numBits=numBitsRM  RMAttribute=RMAttribute  tti=tti  errorCorr=errorCorr  posTrCh=posTrCh  slotFormat=slotFormat  numPhCH=numPhCH  checkRM=off
  Wcdma Rate Matching1 : wcdma_lib/Wcdma Multiplexing and Channel Coding/Wcdma Rate Matching  idxTrCh=2  numBits=numBitsRM  RMAttribute=RMAttribute  tti=tti  errorCorr=errorCorr  posTrCh=posTrCh  slotFormat=slotFormat  numPhCH=numPhCH  checkRM=off
  TrChOut1 : Outport
  TrChOut2 : Outport  Port=2
  wires:
  TrChIn1/1 -> Wcdma Rate Matching/1
  TrChIn2/1 -> Wcdma Rate Matching1/1
  Wcdma Rate Matching/1 -> TrChOut1/1
  Wcdma Rate Matching1/1 -> TrChOut2/1

== system wcdma_lib/Wcdma Multiplexing and Channel Coding/Syndrome Dectector ==
  TrChIn1 : Inport  LatchInput=off
  TrChIn2 : Inport  Port=2  LatchInput=off
  Wcdma CRC Syndrome Detector : wcdma_lib/Wcdma Multiplexing and Channel Coding/Wcdma CRC Syndrome Detector  bits=crcSize(1)  iniStates=0  dataFrames=numTrBlks(1)
  Wcdma CRC Syndrome Detector1 : wcdma_lib/Wcdma Multiplexing and Channel Coding/Wcdma CRC Syndrome Detector  bits=crcSize(2)  iniStates=0  dataFrames=numTrBlks(2)
  TrChOut1 : Outport
  BLER1 : Outport  Port=2
  TrChOut2 : Outport  Port=3
  BLER2 : Outport  Port=4
  wires:
  Wcdma CRC Syndrome Detector/1 -> TrChOut1/1
  TrChIn1/1 -> Wcdma CRC Syndrome Detector/1
  Wcdma CRC Syndrome Detector/2 -> BLER1/1
  Wcdma CRC Syndrome Detector1/1 -> TrChOut2/1
  TrChIn2/1 -> Wcdma CRC Syndrome Detector1/1
  Wcdma CRC Syndrome Detector1/2 -> BLER2/1

== system wcdma_lib/Wcdma Multiplexing and Channel Coding/TrBlk Concatenat Code Blk Segment ==
  TrChIn1 : Inport  LatchInput=off
  TrChIn2 : Inport  Port=2  LatchInput=off
  Concatenation : dspbuff3/Buffer  N=numBitsTrCh(1)  V=0  ic=0
  Concatenation1 : dspbuff3/Buffer  N=numBitsTrCh(2)  V=0  ic=0
  Flip{,1..3} (4 alike) : dspindex/Flip  dim=Columns
  Pad : dspsigops/Pad  padVal=0  padAlong=Columns  numOutRows=numBitsTrCh(1)+numPadBits(1)  numOutCols=1  trunc_flag=None
  Pad1 : dspsigops/Pad  padVal=0  padAlong=Columns  numOutRows=numBitsTrCh(2)+numPadBits(2)  numOutCols=1  trunc_flag=None
  Segmentation1 : dspbuff3/Buffer  N=numBitsCodeWord(1)  V=0  ic=0
  Segmentation2 : dspbuff3/Buffer  N=numBitsCodeWord(2)  V=0  ic=0
  TrChOut1 : Outport
  TrChOut2 : Outport  Port=2
  wires:
  Flip3/1 -> Segmentation2/1
  Flip2/1 -> Pad1/1
  Flip1/1 -> Segmentation1/1
  Flip/1 -> Pad/1
  TrChIn1/1 -> Concatenation/1
  TrChIn2/1 -> Concatenation1/1
  Concatenation/1 -> Flip/1
  Segmentation1/1 -> TrChOut1/1
  Concatenation1/1 -> Flip2/1
  Segmentation2/1 -> TrChOut2/1
  Pad/1 -> Flip1/1
  Pad1/1 -> Flip3/1

== system wcdma_lib/Wcdma Multiplexing and Channel Coding/Wcdma 1st DeInterleaver ==
  In1 : Inport  LatchInput=off
  General Block Deinterleaver : commblkintrlv2/General Block Deinterleaver  elements=int_table
  Out1 : Outport
  wires:
  In1/1 -> General Block Deinterleaver/1
  General Block Deinterleaver/1 -> Out1/1

== system wcdma_lib/Wcdma Multiplexing and Channel Coding/Wcdma 1st Interleaver ==
  In1 : Inport  LatchInput=off
  General Block Interleaver : commblkintrlv2/General Block Interleaver  elements=int_table
  Out1 : Outport
  wires:
  General Block Interleaver/1 -> Out1/1
  In1/1 -> General Block Interleaver/1

== system wcdma_lib/Wcdma Multiplexing and Channel Coding/Wcdma 2nd DeInterleaver ==
  In1 : Inport  LatchInput=off
  General Block Deinterleaver : commblkintrlv2/General Block Deinterleaver  elements=int_table
  Out1 : Outport
  wires:
  General Block Deinterleaver/1 -> Out1/1
  In1/1 -> General Block Deinterleaver/1

== system wcdma_lib/Wcdma Multiplexing and Channel Coding/Wcdma 2nd Interleaver ==
  In1 : Inport  LatchInput=off
  General Block Interleaver : commblkintrlv2/General Block Interleaver  elements=int_table
  Out1 : Outport
  wires:
  In1/1 -> General Block Interleaver/1
  General Block Interleaver/1 -> Out1/1

== system wcdma_lib/Wcdma Multiplexing and Channel Coding/Wcdma Channel Decoding ==
  note: No Coding
  note: Convolutional
      | Encoding
  note: Turbocoding
  CodeWordIn : Inport  LatchInput=off
  Bipolar to Unipolar Converter : commutil2/Bipolar to Unipolar Converter  M=2  polarity=Negative
  DSP Constant : dspsrcs4/DSP Constant  Value=enableEnc  SampleMode=Discrete  discreteOutput=Sample-based  continuousOutput=Sample-based  sampTime=tti*(1e-3)  framePeriod=tti*(1e-3)  dataType=Inherit from 'Constant value'  wordLen=16  udDataType=sfix(16)  fracBitsMode=Best precision  numFracBits=15  InterpretAs1D=off  Ts=tti*(1e-3)  FramebasedOutput=off
  Matrix Concatenation : simulink/Math Operations/Matrix Concatenation  numInports=3  catMethod=Vertical
  Multiport Selector : dspindex/Multiport Selector  rowsOrCols=Rows  idxCellArray=selectBits  idxErrMode=Clip Index
  Wcdma Conv Decoding : wcdma_lib/Wcdma Multiplexing and Channel Coding/Wcdma Conv Decoding  errorCorr=errorCorr  numBitsCodeWord=numBitsCodeWord  numCodeWords=numCodeWords
  Zero-Order Hold : ZeroOrderHold  SampleTime=(tti*1e-3)/numCodeWords
  Zero-Order Hold1 : ZeroOrderHold  SampleTime=(tti*1e-3)/numCodeWords
  TrChOut : Outport
  wires:
  CodeWordIn/1 -> Wcdma Conv Decoding/1, Zero-Order Hold1/1, Bipolar to Unipolar Converter/1
  Wcdma Conv Decoding/1 -> Matrix Concatenation/2
  Matrix Concatenation/1 -> Multiport Selector/1
  Multiport Selector/1 -> TrChOut/1
  DSP Constant/1 -> Wcdma Conv Decoding/Enable
  Zero-Order Hold/1 -> Matrix Concatenation/1
  Zero-Order Hold1/1 -> Matrix Concatenation/3
  Bipolar to Unipolar Converter/1 -> Zero-Order Hold/1

== system wcdma_lib/Wcdma Multiplexing and Channel Coding/Wcdma Channel Encoding ==
  note: No Coding
  note: Convolutional Encoding
  note: Turbocoding
  CodeWordIn : Inport  LatchInput=off
  DSP Constant : dspsrcs4/DSP Constant  Value=enableEnc  InterpretAs1D=off  SampleMode=Discrete  Ts=(tti*1e-3)  FramebasedOutput=off
  Matrix Concatenation : simulink3/Signals & Systems/Matrix Concatenation  numInports=3  catMethod=Vertical
  Multiport Selector : dspindex/Multiport Selector  rowsOrCols=Rows  idxCellArray=selectBits  idxErrMode=Clip Index
  Wcdma Conv Encoding : wcdma_lib/Wcdma Multiplexing and Channel Coding/Wcdma Conv Encoding  errorCorr=errorCorr  numBitsCodeWord=numBitsCodeWord  numCodeWords=numCodeWords
  Zero-Order Hold : ZeroOrderHold  SampleTime=tti*1e-3
  Zero-Order Hold1 : ZeroOrderHold  SampleTime=tti*1e-3
  TrChOut : Outport
  wires:
  CodeWordIn/1 -> Wcdma Conv Encoding/1, Zero-Order Hold/1, Zero-Order Hold1/1
  Matrix Concatenation/1 -> Multiport Selector/1
  Multiport Selector/1 -> TrChOut/1
  Wcdma Conv Encoding/1 -> Matrix Concatenation/2
  DSP Constant/1 -> Wcdma Conv Encoding/Enable
  Zero-Order Hold/1 -> Matrix Concatenation/1
  Zero-Order Hold1/1 -> Matrix Concatenation/3

== system wcdma_lib/Wcdma Multiplexing and Channel Coding/Wcdma Turbo DeInterleaver ==
  In1 : Inport  LatchInput=off
  General Block Deinterleaver : commblkintrlv2/General Block Deinterleaver  elements=int_table
  Out1 : Outport
  wires:
  In1/1 -> General Block Deinterleaver/1
  General Block Deinterleaver/1 -> Out1/1

== system wcdma_lib/Wcdma Multiplexing and Channel Coding/Wcdma Turbo Interleaver ==
  In1 : Inport  LatchInput=off
  General Block Interleaver : commblkintrlv2/General Block Interleaver  elements=int_table
  Out1 : Outport
  wires:
  General Block Interleaver/1 -> Out1/1
  In1/1 -> General Block Interleaver/1

== system wcdma_lib/Wcdma Multiplexing and Channel Coding/Wcdma CRC Generator ==
  In : Inport  LatchInput=off
  General CRC Generator : commcrc2/General CRC Generator  genPoly=genPoly  iniStates=iniStates  numChecksums=dataFrames
  Out : Outport
  wires:
  In/1 -> General CRC Generator/1
  General CRC Generator/1 -> Out/1

== system wcdma_lib/Wcdma Multiplexing and Channel Coding/Wcdma CRC Syndrome Detector ==
  In1 : Inport  LatchInput=off
  General CRC Syndrome Detector : commcrc2/General CRC Syndrome Detector  genPoly=genPoly  iniStates=iniStates  numChecksums=dataFrames
  Out1 : Outport
  Out2 : Outport  Port=2
  wires:
  General CRC Syndrome Detector/2 -> Out2/1
  General CRC Syndrome Detector/1 -> Out1/1
  In1/1 -> General CRC Syndrome Detector/1

== system wcdma_lib/Wcdma Multiplexing and Channel Coding/Wcdma Conv Decoding ==
  In1 : Inport  LatchInput=off
  Enable : EnablePort
  Segmentation : dspbuff3/Buffer  N=codeRate*(numBitsCodeWord+tailBits)  V=0  ic=0
  Viterbi Decoder : commcnvcod2/Viterbi Decoder  trellis=trellis  dectype=Unquantized  nsdecb=4  tbdepth=5*8  opmode=Truncated  reset=off
  Zero Pad : dspsigops/Zero Pad  zpadAlong=Columns  numOutRows=numBitsCodeWord  numOutCols=1  trunc_flag=None
  Out1 : Outport
  wires:
  Zero Pad/1 -> Out1/1
  In1/1 -> Segmentation/1
  Segmentation/1 -> Viterbi Decoder/1
  Viterbi Decoder/1 -> Zero Pad/1

== system wcdma_lib/Wcdma Multiplexing and Channel Coding/Wcdma Conv Encoding ==
  In1 : Inport  LatchInput=off
  Enable : EnablePort
  Convolutional Encoder : commcnvcod2/Convolutional Encoder  trellis=trellis  reset=None
  Segmentation : dspbuff3/Buffer  N=codeRate*(numBitsCodeWord+tailBits)*numCodeWords  V=0  ic=0
  Zero Pad1 : dspsigops/Zero Pad  zpadAlong=Columns  numOutRows=numBitsCodeWord+tailBits  numOutCols=1  trunc_flag=None
  Out1 : Outport
  wires:
  Segmentation/1 -> Out1/1
  In1/1 -> Zero Pad1/1
  Zero Pad1/1 -> Convolutional Encoder/1
  Convolutional Encoder/1 -> Segmentation/1

== system wcdma_lib/Wcdma Multiplexing and Channel Coding/Wcdma Rx Channel Decoding Scheme ==
  note: Wcdma Physical Channel RX Error Correction
  note: Rate
      | DeMatching
  note: 1st
      | Deinterleaver
  note: Channel
      | Decoding
  note: Code Blk Concat/
      |  TrBlk Segm
  note: Syndrome
      | Detector
  note: Radio Frame
      | Concatenation
  CCtrChIn1 : Inport  LatchInput=off
  1st DeInterleaver : wcdma_lib/Wcdma Multiplexing and Channel Coding/1st DeInterleaver
  Channel Decoding : wcdma_lib/Wcdma Multiplexing and Channel Coding/Channel Decoding
  Code Blk Concatenat TrBlk Segment : wcdma_lib/Wcdma Multiplexing and Channel Coding/Code Blk Concatenat TrBlk Segment  trBlkSetSize=trBlkSetSize  trBlkSize=trBlkSize  crcSize=crcSize
  Radio Frame  Concatenation : wcdma_lib/Wcdma Multiplexing and Channel Coding/Radio Frame  Concatenation  numBits=numBitsFirstInt  tti=tti  checkDelay=on
  Rate DeMatching : wcdma_lib/Wcdma Multiplexing and Channel Coding/Rate DeMatching
  Syndrome Dectector : wcdma_lib/Wcdma Multiplexing and Channel Coding/Syndrome Dectector
  background6 : Subsystem  EnableExecutionContextPropagation=on
      mask Display: disp('')
  TrChOut1 : Outport
  BLER1 : Outport  Port=2
  TrChOut3 : Outport  Port=3
  BLER2 : Outport  Port=4
  wires:
  1st DeInterleaver/1 -> Rate DeMatching/1  "dtch"
  1st DeInterleaver/2 -> Rate DeMatching/2  "dcch"
  Rate DeMatching/1 -> Channel Decoding/1  "dtch"
  Rate DeMatching/2 -> Channel Decoding/2  "dcch"
  Channel Decoding/1 -> Code Blk Concatenat TrBlk Segment/1  "dtch"
  Channel Decoding/2 -> Code Blk Concatenat TrBlk Segment/2  "dcch"
  Code Blk Concatenat TrBlk Segment/1 -> Syndrome Dectector/1  "dtch"
  Code Blk Concatenat TrBlk Segment/2 -> Syndrome Dectector/2  "dcch"
  Syndrome Dectector/1 -> TrChOut1/1  "dtch"
  Syndrome Dectector/2 -> BLER1/1  "syn1"
  Syndrome Dectector/3 -> TrChOut3/1  "dcch"
  Syndrome Dectector/4 -> BLER2/1  "syn2"
  CCtrChIn1/1 -> Radio Frame  Concatenation/1  "cctrch"
  Radio Frame  Concatenation/1 -> 1st DeInterleaver/1  "dtch"
  Radio Frame  Concatenation/2 -> 1st DeInterleaver/2  "dcch"

== system wcdma_lib/Wcdma Multiplexing and Channel Coding/Wcdma Rx PhCh Demapping ==
  note: Wcdma Rx Physical Channel Demapping
  note: Ph Channel
      | Demapping
  note: 2nd
      | Deinterleaver
  note: Ph Channel
      | Concatenation
  note: Slot
      | Splitter
  PhChIn1 : Inport  LatchInput=off
  2nd DeInterleaver : wcdma_lib/Wcdma Multiplexing and Channel Coding/2nd DeInterleaver
  PhCh Concatenation : wcdma_lib/Wcdma Multiplexing and Channel Coding/PhCh Concatenation
  TPC Bits : Terminator
  Wcdma Slot  Splitter : wcdma_lib/Wcdma Multiplexing and Channel Coding/Wcdma Slot  Splitter  slotFormat=slotFormat  numSlotDelay=3
  background6 : Subsystem  EnableExecutionContextPropagation=on
      mask Display: disp('')
  CCTrChOut1 : Outport
  wires:
  2nd DeInterleaver/1 -> PhCh Concatenation/1  "cctrch"
  PhCh Concatenation/1 -> CCTrChOut1/1  "cctrch"
  Wcdma Slot  Splitter/1 -> 2nd DeInterleaver/1
  PhChIn1/1 -> Wcdma Slot  Splitter/1  "slot"
  Wcdma Slot  Splitter/2 -> TPC Bits/1

== system wcdma_lib/Wcdma Multiplexing and Channel Coding/Wcdma Slot  Builder ==
  PhChIn1 : Inport  LatchInput=off
  TPCBits : Inport  Port=2  LatchInput=off
  Buffer : dspbuff3/Buffer  N=Ndata1+Ndata2  V=0  ic=0
  Matrix Concatenation : simulink/Math Operations/Matrix Concatenation  numInports=5  catMethod=Vertical
  Multiport Selector1 : dspindex/Multiport Selector  rowsOrCols=Rows  idxCellArray={[1:Ndata1prima] [Ndata1+1:Ndata1+Ndata2] }  idxErrMode=Clip and Warn
  Puncture : commsequence2/Puncture  punctureVector=punctPattern
  Repeat : dspsigops/Repeat  N=Ntpc  ic=0  mode=Maintain input frame rate
  TFCI Bits : dspsrcs4/DSP Constant  Value=ones(Ntfciprima,1)  SampleMode=Discrete  discreteOutput=Frame-based  continuousOutput=Sample-based  sampTime=0.01/15  framePeriod=0.01/15  dataType=Inherit from 'Constant value'  wordLen=16  udDataType=sfix(16)  fracBitsMode=Best precision  numFracBits=15  InterpretAs1D=off  Ts=0.01/15  FramebasedOutput=on
  Wcdma Pilot Bits Generator : wcdma_lib/Wcdma Sources/Wcdma Pilot Bits Generator  numPilotBits=Npilot  frameSampTime=0.01
  PhChOut1 : Outport
  wires:
  PhChIn1/1 -> Buffer/1  "DPCH"
  Multiport Selector1/1 -> Matrix Concatenation/1  "Data1"
  Matrix Concatenation/1 -> Puncture/1
  TPCBits/1 -> Repeat/1
  Repeat/1 -> Matrix Concatenation/2  "TPC"
  TFCI Bits/1 -> Matrix Concatenation/3  "TFCI"
  Multiport Selector1/2 -> Matrix Concatenation/4  "Data2"
  Wcdma Pilot Bits Generator/1 -> Matrix Concatenation/5  "Pilot Bits"
  Buffer/1 -> Multiport Selector1/1
  Puncture/1 -> PhChOut1/1  "Slot"

== system wcdma_lib/Wcdma Multiplexing and Channel Coding/Wcdma Slot  Splitter ==
  PhChIn1 : Inport  LatchInput=off
  Buffer : dspbuff3/Buffer  N=(Ndata1+Ndata2)*15  V=0  ic=0
  Delay : dspsigops/Delay  dly_unit=Samples  delay=(Ndata1+Ndata2)*15-samplesDelay  ic_detail=off  dif_ic_for_ch=off  dif_ic_for_dly=off  ic=0  reset_popup=None
  Matrix Concatenation : simulink/Math Operations/Matrix Concatenation  numInports=2  catMethod=Vertical
  Mean : dspstat3/Mean  run=off  reset_popup=None
  Multiport Selector : S-Function  FunctionName=sdspmultiportsel  Parameters=rowsOrCols, numOutports, flatIdxVect, flatLenVect, idxErrMode  mask(Multiport Selector){rowsOrCols=Rows, idxCellArray=selectPattern2, idxErrMode=Clip and Warn}
      mask prompts: rowsOrCols "Select:"; idxCellArray "Indices to output:"; idxErrMode "Invalid index:"
      mask help: Output specified rows or columns to one or more output ports. The number of output ports is determined by the number of index vectors, each specified as a separate vector entry in a cell array. Indices are 1-based and need not be unique.
      mask init:
      | [numOutports, flatLenVect, flatIdxVect] = dspblkmultiportsel(idxCellArray);
      mask Help: web(dspbhelp);
      mask StyleString: popup(Rows|Columns),edit,popup(Clip Index|Clip and Warn|Generate Error)
      mask Display: disp(['Select\n' &1]);
  Multiport Selector1 : S-Function  FunctionName=sdspmultiportsel  Parameters=rowsOrCols, numOutports, flatIdxVect, flatLenVect, idxErrMode  mask(Multiport Selector){rowsOrCols=Rows, idxCellArray=selectPattern, idxErrMode=Clip and Warn}
      mask prompts: rowsOrCols "Select:"; idxCellArray "Indices to output:"; idxErrMode "Invalid index:"
      mask help: Output specified rows or columns to one or more output ports. The number of output ports is determined by the number of index vectors, each specified as a separate vector entry in a cell array. Indices are 1-based and need not be unique.
      mask init:
      | [numOutports, flatLenVect, flatIdxVect] = dspblkmultiportsel(idxCellArray);
      mask Help: web(dspbhelp);
      mask StyleString: popup(Rows|Columns),edit,popup(Clip Index|Clip and Warn|Generate Error)
      mask Display: disp('Slot\nSplitter');
  Terminator1 : Terminator
  Terminator2 : Terminator
  PhChOut1 : Outport
  PhChOut2 : Outport  Port=2
  wires:
  PhChIn1/1 -> Multiport Selector1/1  "Slot"
  Multiport Selector1/1 -> Matrix Concatenation/1  "Data1"
  Matrix Concatenation/1 -> Multiport Selector/1
  Buffer/1 -> PhChOut1/1  "DPCH"
  Multiport Selector1/2 -> Mean/1  "TPC"
  Mean/1 -> PhChOut2/1
  Multiport Selector1/3 -> Terminator1/1  "TFCI"
  Multiport Selector1/4 -> Matrix Concatenation/2  "Data2"
  Multiport Selector/1 -> Delay/1  "Data1 + Data2"
  Multiport Selector1/5 -> Terminator2/1  "Pilot bits"
  Delay/1 -> Buffer/1

== system wcdma_lib/Wcdma Multiplexing and Channel Coding/Wcdma Tx PhCh Mapping ==
  note: Wcdma Tx Physical Channel Mapping
  note: Ph Channel
      | Segmentation
  note: 2nd
      | Interleaver
  note: Ph Channel
      | Mapping
  note: Slot Builder
  CCTrChIn1 : Inport  LatchInput=off
  2nd Interleaver : wcdma_lib/Wcdma Multiplexing and Channel Coding/2nd Interleaver
  PhCh Segmentation : wcdma_lib/Wcdma Multiplexing and Channel Coding/PhCh Segmentation
  TPC Bits : dspsrcs4/DSP Constant  Value=1  InterpretAs1D=off  SampleMode=Discrete  Ts=0.01/15  FramebasedOutput=on
  Wcdma Slot  Builder : wcdma_lib/Wcdma Multiplexing and Channel Coding/Wcdma Slot  Builder  slotFormat=slotFormat
  background6 : Subsystem  EnableExecutionContextPropagation=on
      mask Display: disp('')
  PhChOut1 : Outport
  wires:
  PhCh Segmentation/1 -> 2nd Interleaver/1  "phch"
  2nd Interleaver/1 -> Wcdma Slot  Builder/1
  CCTrChIn1/1 -> PhCh Segmentation/1  "cctrch"
  Wcdma Slot  Builder/1 -> PhChOut1/1  "slot"
  TPC Bits/1 -> Wcdma Slot  Builder/2
